simulink model "xfl_ukf2"  (R2015b)
settings: Solver=FixedStepAuto  StartTime=0  StopTime=5  FixedStep=10*(1e-3)  RelTol=1e-3
undefined symbols (not defined in the file or in its folder): qc
libraries: simulink x2
settings Model: Creator=acsl  LastModifiedBy=acsl

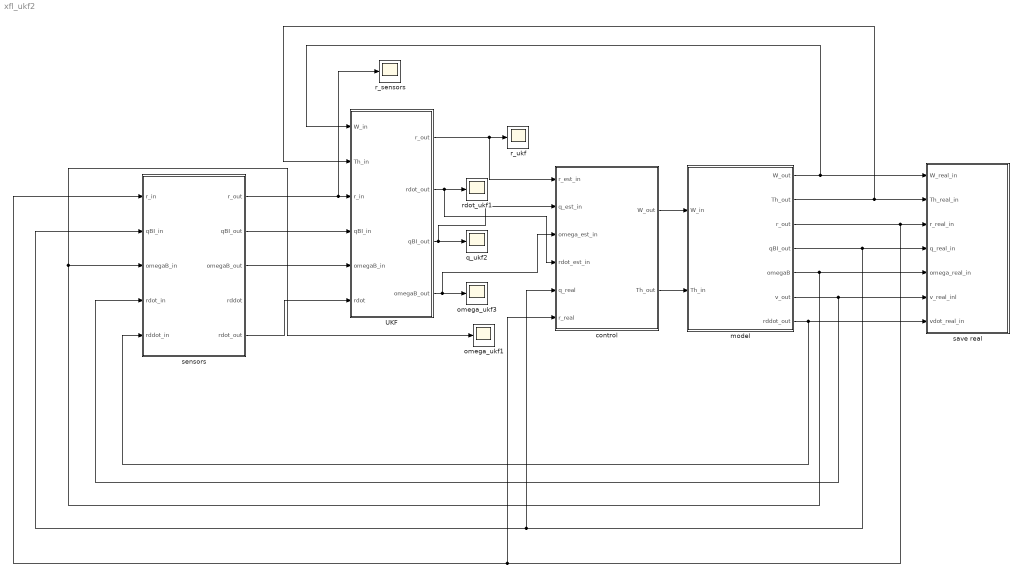
== system xfl_ukf2 ==
  UKF : Subsystem
  control : Subsystem  InitFcn=init
  model : Subsystem
  omega_ukf1 : Scope
  omega_ukf3 : Scope
  q_ukf2 : Scope
  r_sensors : Scope
  r_ukf : Scope
  rdot_ukf1 : Scope
  save real : Subsystem
  sensors : Subsystem
  wires:
  model/2(Th_out) -> UKF/2(Th_in), save real/2(Th_real_in)
  model/7(rddot_out) -> sensors/5(rddot_in), save real/7(vdot_real_in)
  model/5(omegaB) -> sensors/3(omegaB_in), omega_ukf1/1, save real/5(omega_real_in)
  control/1(W_out) -> model/1(W_in)
  control/2(Th_out) -> model/2(Th_in)
  model/3(r_out) -> control/6(r_real), sensors/1(r_in), save real/3(r_real_in)
  model/4(qBI_out) -> sensors/2(qBI_in), control/5(q_real), save real/4(q_real_in)
  model/6(v_out) -> sensors/4(rdot_in), save real/6(v_real_inl)
  model/1(W_out) -> UKF/1(W_in), save real/1(W_real_in)
  sensors/3(omegaB_out) -> UKF/5(omegaB_in)
  sensors/2(qBI_out) -> UKF/4(qBI_in)
  sensors/1(r_out) -> r_sensors/1, UKF/3(r_in)
  UKF/2(rdot_out) -> rdot_ukf1/1, control/4(rdot_est_in)
  UKF/3(qBI_out) -> control/2(q_est_in), q_ukf2/1
  UKF/4(omegaB_out) -> control/3(omega_est_in), omega_ukf3/1
  UKF/1(r_out) -> r_ukf/1, control/1(r_est_in)
  sensors/5(rdot_out) -> UKF/6(rdot)

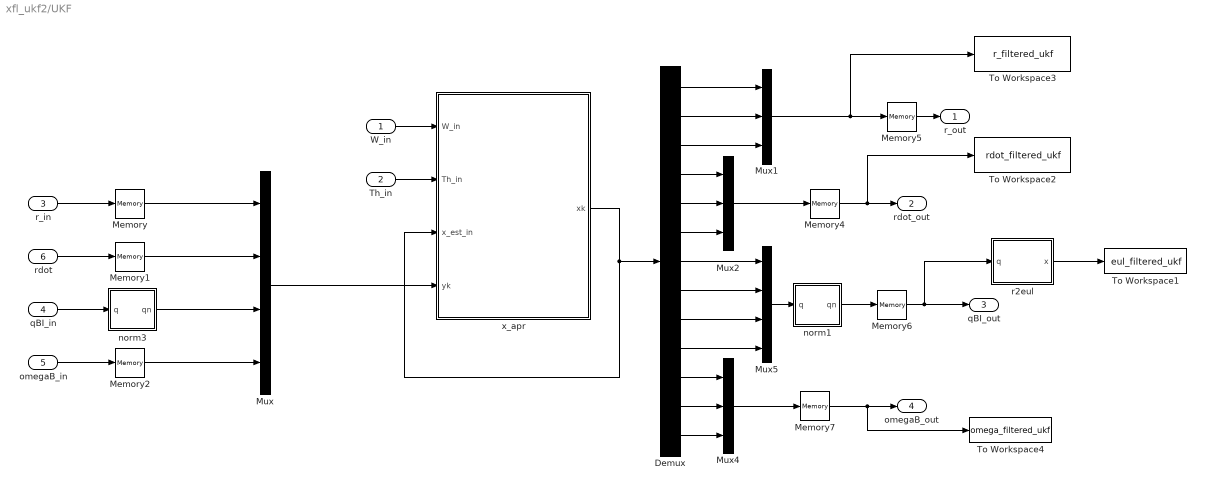
== system xfl_ukf2/UKF ==
  W_in : Inport
  Th_in : Inport  Port=2
  r_in : Inport  Port=3
  qBI_in : Inport  Port=4
  omegaB_in : Inport  Port=5
  rdot : Inport  Port=6
  Demux : Demux  Outputs=13
  Memory : Memory  X0=qc.r0
  Memory{1..2,4,7} (4 alike) : Memory  X0=[0 0 0]'
  Memory5 : Memory  X0=qc.r0
  Memory6 : Memory  X0=qc.qBI0
  Mux : Mux
  Mux1 : Mux  Inputs=3
  Mux2 : Mux  Inputs=3
  Mux4 : Mux  Inputs=3
  Mux5 : Mux
  To Workspace1 : ToWorkspace  VariableName=eul_filtered_ukf  SaveFormat=Timeseries  SampleTime=-1
  To Workspace2 : ToWorkspace  VariableName=rdot_filtered_ukf  SaveFormat=Timeseries  SampleTime=-1
  To Workspace3 : ToWorkspace  VariableName=r_filtered_ukf  SaveFormat=Timeseries  SampleTime=-1
  To Workspace4 : ToWorkspace  VariableName=omega_filtered_ukf  SaveFormat=Timeseries  SampleTime=-1
  norm1 : MATLAB Function  TreatAsAtomicUnit=on
  norm3 : MATLAB Function  TreatAsAtomicUnit=on
  r2eul : MATLAB Function  TreatAsAtomicUnit=on
  x_apr : Subsystem
  r_out : Outport
  rdot_out : Outport  Port=2
  qBI_out : Outport  Port=3
  omegaB_out : Outport  Port=4
  wires:
  qBI_in/1 -> norm3/1(q)
  omegaB_in/1 -> Memory2/1
  rdot/1 -> Memory1/1
  W_in/1 -> x_apr/1(W_in)
  Th_in/1 -> x_apr/2(Th_in)
  Demux/1 -> Mux1/1
  Demux/2 -> Mux1/2
  Demux/3 -> Mux1/3
  Demux/4 -> Mux2/1
  Demux/6 -> Mux2/3
  Demux/5 -> Mux2/2
  Demux/9 -> Mux5/3
  Demux/7 -> Mux5/1
  Demux/8 -> Mux5/2
  Demux/11 -> Mux4/1
  Demux/12 -> Mux4/2
  Demux/13 -> Mux4/3
  Demux/10 -> Mux5/4
  Mux1/1 -> To Workspace3/1, Memory5/1
  Mux2/1 -> Memory4/1
  Mux5/1 -> norm1/1(q)
  r_in/1 -> Memory/1
  norm1/1(qn) -> Memory6/1
  Mux4/1 -> Memory7/1
  r2eul/1(x) -> To Workspace1/1
  Mux/1 -> x_apr/4(yk)
  x_apr/1(xk) -> Demux/1, x_apr/3(x_est_in)
  Memory/1 -> Mux/1
  Memory1/1 -> Mux/2
  Memory2/1 -> Mux/4
  norm3/1(qn) -> Mux/3
  Memory5/1 -> r_out/1
  Memory4/1 -> To Workspace2/1, rdot_out/1
  Memory6/1 -> r2eul/1(q), qBI_out/1
  Memory7/1 -> To Workspace4/1, omegaB_out/1

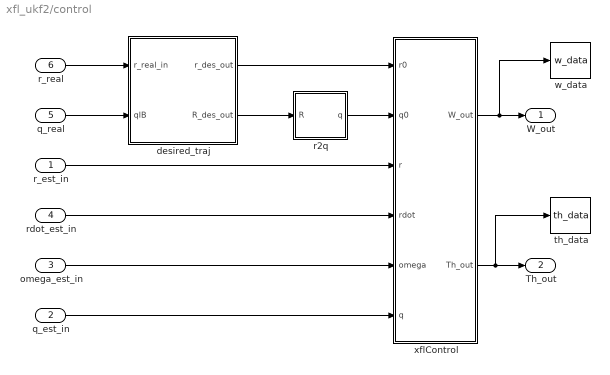
== system xfl_ukf2/control ==
  r_est_in : Inport
  q_est_in : Inport  Port=2
  omega_est_in : Inport  Port=3
  rdot_est_in : Inport  Port=4
  q_real : Inport  Port=5
  r_real : Inport  Port=6
  desired_traj : Subsystem
  r2q : MATLAB Function  TreatAsAtomicUnit=on
  th_data : ToWorkspace  VariableName=th_data  SaveFormat=Timeseries  SampleTime=-1
  w_data : ToWorkspace  VariableName=w_data  SaveFormat=Timeseries  SampleTime=-1
  xflControl : Subsystem
  W_out : Outport
  Th_out : Outport  Port=2
  wires:
  omega_est_in/1 -> xflControl/5(omega)
  q_est_in/1 -> xflControl/6(q)
  rdot_est_in/1 -> xflControl/4(rdot)
  r_est_in/1 -> xflControl/3(r)
  desired_traj/1(r_des_out) -> xflControl/1(r0)
  desired_traj/2(R_des_out) -> r2q/1(R)
  xflControl/1(W_out) -> w_data/1, W_out/1
  xflControl/2(Th_out) -> th_data/1, Th_out/1
  r2q/1(q) -> xflControl/2(q0)
  r_real/1 -> desired_traj/1(r_real_in)
  q_real/1 -> desired_traj/2(qIB)

== system xfl_ukf2/model ==
  W_in : Inport
  Th_in : Inport  Port=2
  draw : Subsystem
  dynamic : Subsystem  StopFcn=close all
  integration : Subsystem
  W_out : Outport
  Th_out : Outport  Port=2
  r_out : Outport  Port=3
  qBI_out : Outport  Port=4
  omegaB : Outport  Port=5
  v_out : Outport  Port=6
  rddot_out : Outport  Port=7
  wires:
  integration/1(r_out) -> dynamic/3(r_in), r_out/1
  dynamic/2(F_I_out) -> integration/2(F_B_in)
  integration/2(qBI_out) -> dynamic/4(q_BI_in), draw/2(qBI), qBI_out/1
  W_in/1 -> W_out/1, dynamic/1(W_in)
  dynamic/1(tau_B_out) -> integration/1(tau_in)
  integration/3(omegaB_out) -> dynamic/5(omegaB_in), omegaB/1
  Th_in/1 -> dynamic/2(Th_in), Th_out/1
  dynamic/3(q_PB_out) -> draw/1(q_PB)
  integration/4(v_out) -> v_out/1
  integration/5(rddot_out) -> rddot_out/1

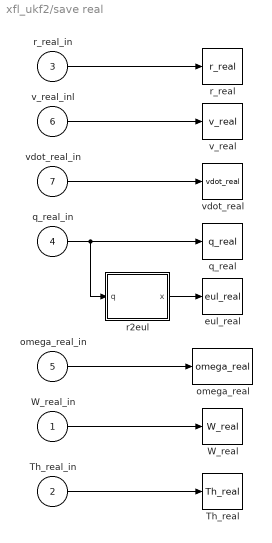
== system xfl_ukf2/save real ==
  W_real_in : Inport
  Th_real_in : Inport  Port=2
  r_real_in : Inport  Port=3
  q_real_in : Inport  Port=4
  omega_real_in : Inport  Port=5
  v_real_inl : Inport  Port=6
  vdot_real_in : Inport  Port=7
  Th_real : ToWorkspace  VariableName=Th_real  SaveFormat=Timeseries  SampleTime=-1
  W_real : ToWorkspace  VariableName=W_real  SaveFormat=Timeseries  SampleTime=-1
  eul_real : ToWorkspace  VariableName=eul_real  SaveFormat=Timeseries  SampleTime=-1
  omega_real : ToWorkspace  VariableName=omega_real  SaveFormat=Timeseries  SampleTime=-1
  q_real : ToWorkspace  VariableName=q_real  SaveFormat=Timeseries  SampleTime=-1
  r2eul : MATLAB Function  TreatAsAtomicUnit=on
  r_real : ToWorkspace  VariableName=r_real  SaveFormat=Timeseries  SampleTime=-1
  v_real : ToWorkspace  VariableName=v_real  SaveFormat=Timeseries  SampleTime=-1
  vdot_real : ToWorkspace  VariableName=vdot_real  SaveFormat=Timeseries  SampleTime=-1
  wires:
  q_real_in/1 -> q_real/1, r2eul/1(q)
  r_real_in/1 -> r_real/1
  v_real_inl/1 -> v_real/1
  vdot_real_in/1 -> vdot_real/1
  r2eul/1(x) -> eul_real/1
  omega_real_in/1 -> omega_real/1
  Th_real_in/1 -> Th_real/1
  W_real_in/1 -> W_real/1

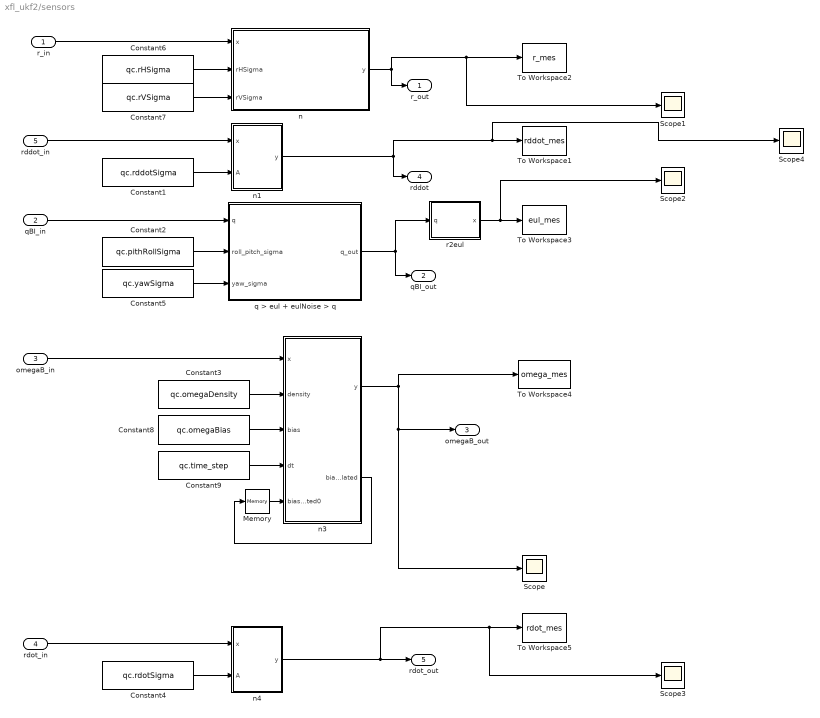
== system xfl_ukf2/sensors ==
  r_in : Inport
  qBI_in : Inport  Port=2
  omegaB_in : Inport  Port=3
  rdot_in : Inport  Port=4
  rddot_in : Inport  Port=5
  Constant1 : Constant  Value=qc.rddotSigma
  Constant2 : Constant  Value=qc.pithRollSigma
  Constant3 : Constant  Value=qc.omegaDensity
  Constant4 : Constant  Value=qc.rdotSigma
  Constant5 : Constant  Value=qc.yawSigma
  Constant6 : Constant  Value=qc.rHSigma
  Constant7 : Constant  Value=qc.rVSigma
  Constant8 : Constant  Value=qc.omegaBias
  Constant9 : Constant  Value=qc.time_step
  Memory : Memory  X0=[0;0;0]
  Scope{,1..4} (5 alike) : Scope
  To Workspace1 : ToWorkspace  VariableName=rddot_mes  SaveFormat=Timeseries  SampleTime=-1
  To Workspace2 : ToWorkspace  VariableName=r_mes  SaveFormat=Timeseries  SampleTime=-1
  To Workspace3 : ToWorkspace  VariableName=eul_mes  SaveFormat=Timeseries  SampleTime=-1
  To Workspace4 : ToWorkspace  VariableName=omega_mes  SaveFormat=Timeseries  SampleTime=-1
  To Workspace5 : ToWorkspace  VariableName=rdot_mes  SaveFormat=Timeseries  SampleTime=-1
  n : MATLAB Function  TreatAsAtomicUnit=on
  n1 : MATLAB Function  TreatAsAtomicUnit=on
  n3 : MATLAB Function  TreatAsAtomicUnit=on
  n4 : MATLAB Function  TreatAsAtomicUnit=on
  q > eul + eulNoise > q : MATLAB Function  TreatAsAtomicUnit=on
  r2eul : MATLAB Function  TreatAsAtomicUnit=on
  r_out : Outport
  qBI_out : Outport  Port=2
  omegaB_out : Outport  Port=3
  rddot : Outport  Port=4
  rdot_out : Outport  Port=5
  wires:
  rddot_in/1 -> n1/1(x)
  qBI_in/1 -> q > eul + eulNoise > q/1(q)
  n3/1(y) -> omegaB_out/1, Scope/1, To Workspace4/1
  q > eul + eulNoise > q/1(q_out) -> qBI_out/1, r2eul/1(q)
  n/1(y) -> Scope1/1, To Workspace2/1, r_out/1
  n1/1(y) -> Scope4/1, To Workspace1/1, rddot/1
  r2eul/1(x) -> Scope2/1, To Workspace3/1
  r_in/1 -> n/1(x)
  Constant6/1 -> n/2(rHSigma)
  Constant1/1 -> n1/2(A)
  Constant2/1 -> q > eul + eulNoise > q/2(roll_pitch_sigma)
  Constant3/1 -> n3/2(density)
  Constant4/1 -> n4/2(A)
  rdot_in/1 -> n4/1(x)
  n4/1(y) -> Scope3/1, To Workspace5/1, rdot_out/1
  Constant5/1 -> q > eul + eulNoise > q/3(yaw_sigma)
  Constant7/1 -> n/3(rVSigma)
  Constant8/1 -> n3/3(bias)
  Constant9/1 -> n3/4(dt)
  Memory/1 -> n3/5(bias_accumulated0)
  n3/2(bias_accumulated) -> Memory/1
  omegaB_in/1 -> n3/1(x)

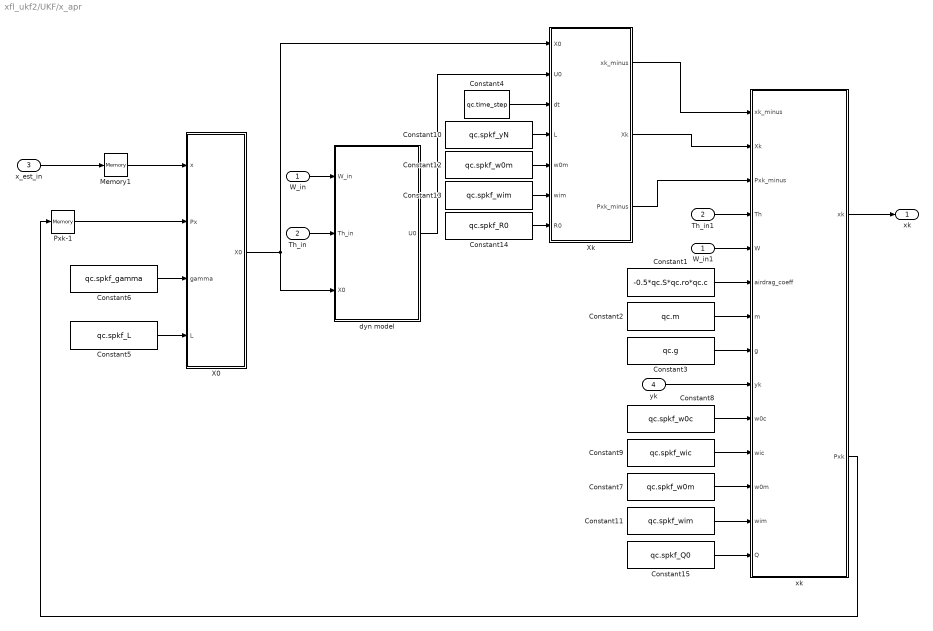
== system xfl_ukf2/UKF/x_apr ==
  W_in : Inport
  Th_in : Inport  Port=2
  x_est_in : Inport  Port=3
  yk : Inport  Port=4
  Constant1 : Constant  Value=-0.5*qc.S*qc.ro*qc.c
  Constant10 : Constant  Value=qc.spkf_yN
  Constant11 : Constant  Value=qc.spkf_wim
  Constant12 : Constant  Value=qc.spkf_w0m
  Constant13 : Constant  Value=qc.spkf_wim
  Constant14 : Constant  Value=qc.spkf_R0
  Constant15 : Constant  Value=qc.spkf_Q0
  Constant2 : Constant  Value=qc.m
  Constant3 : Constant  Value=qc.g
  Constant4 : Constant  Value=qc.time_step
  Constant5 : Constant  Value=qc.spkf_L
  Constant6 : Constant  Value=qc.spkf_gamma
  Constant7 : Constant  Value=qc.spkf_w0m
  Constant8 : Constant  Value=qc.spkf_w0c
  Constant9 : Constant  Value=qc.spkf_wic
  Memory1 : Memory  X0="[0 0 0    0 0 0    1 0 0 0    0 0 0]'"  InheritSampleTime=on
  Pxk-1 : Memory  X0="diag([10 10 10      10 10 10     1e-1 1e-1 1e-1 1e-1    1e-1 1e-1 1e-1])"  InheritSampleTime=on
  Th_in1 : InportShadow  Port=2
  W_in1 : InportShadow
  X0 : MATLAB Function  TreatAsAtomicUnit=on
  Xk : MATLAB Function  TreatAsAtomicUnit=on
  dyn model : Subsystem
  "xk " : MATLAB Function  TreatAsAtomicUnit=on
  xk : Outport
  wires:
  Th_in/1 -> dyn model/2(Th_in)
  W_in/1 -> dyn model/1(W_in)
  x_est_in/1 -> Memory1/1
  Memory1/1 -> X0/1(x)
  X0/1(X0) -> Xk/1(X0), dyn model/3("X0 ")
  dyn model/1(U0) -> Xk/2(U0)
  Constant4/1 -> Xk/3(dt)
  Xk/1(xk_minus) -> "xk "/1(xk_minus)
  Constant1/1 -> "xk "/6(airdrag_coeff)
  Constant2/1 -> "xk "/7(m)
  Constant3/1 -> "xk "/8(g)
  Xk/2(Xk) -> "xk "/2(Xk)
  "xk "/1(xk) -> xk/1
  yk/1 -> "xk "/9(yk)
  Xk/3(Pxk_minus) -> "xk "/3(Pxk_minus)
  Th_in1/1 -> "xk "/4(Th)
  W_in1/1 -> "xk "/5(W)
  Pxk-1/1 -> X0/2(Px)
  "xk "/2(Pxk) -> Pxk-1/1
  Constant5/1 -> X0/4(L)
  Constant6/1 -> X0/3(gamma)
  Constant10/1 -> Xk/4(L)
  Constant12/1 -> Xk/5(w0m)
  Constant13/1 -> Xk/6(wim)
  Constant8/1 -> "xk "/10(w0c)
  Constant9/1 -> "xk "/11(wic)
  Constant7/1 -> "xk "/12(w0m)
  Constant11/1 -> "xk "/13(wim)
  Constant14/1 -> Xk/7(R0)
  Constant15/1 -> "xk "/14(Q)

== system xfl_ukf2/control/desired_traj ==
  r_real_in : Inport
  qIB : Inport  Port=2
  To Workspace1 : ToWorkspace  VariableName=time  SaveFormat=Timeseries  SampleTime=-1
  To Workspace2 : ToWorkspace  VariableName=r_des  SaveFormat=Timeseries  SampleTime=-1
  To Workspace6 : ToWorkspace  VariableName=eul_des  SaveFormat=Timeseries  SampleTime=-1
  dirB : ToWorkspace  VariableName=dirB  SaveFormat=Timeseries  SampleTime=-1
  rFr3 : Scope
  r_target : ToWorkspace  VariableName=r_target  SaveFormat=Timeseries  SampleTime=-1
  time : simulink/Sources/Ramp  slope=1  start=0  X0=0
  traj : MATLAB Function  TreatAsAtomicUnit=on
  r_des_out : Outport
  R_des_out : Outport  Port=2
  wires:
  traj/2(R_des) -> R_des_out/1
  time/1 -> To Workspace1/1, traj/1(t)
  traj/3(eul_des) -> To Workspace6/1
  r_real_in/1 -> traj/2(r)
  traj/1(r_des) -> To Workspace2/1, r_des_out/1
  qIB/1 -> traj/3(qIB)
  traj/4(camera_dir_B) -> dirB/1, rFr3/1
  traj/5(r_target) -> r_target/1

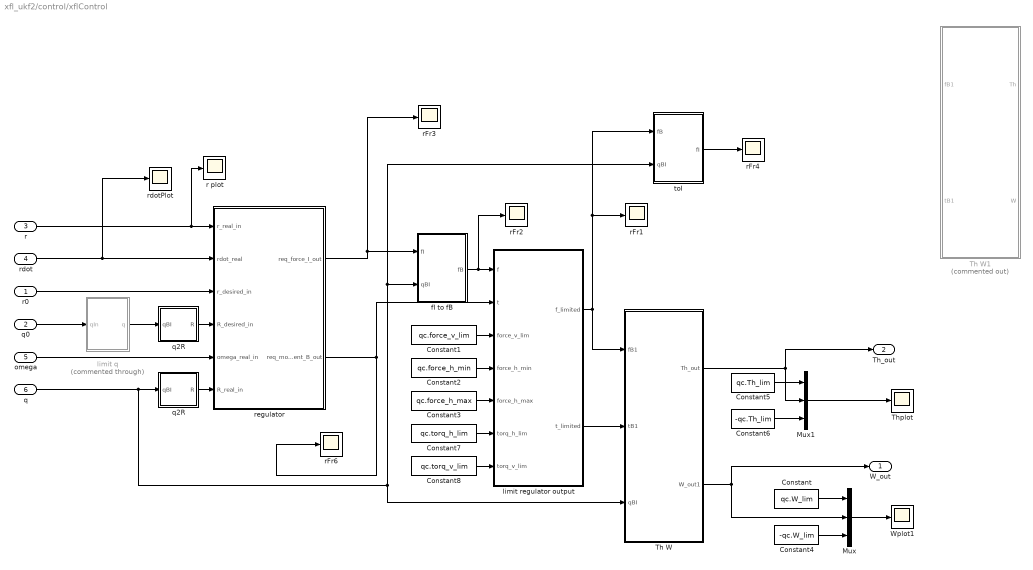
== system xfl_ukf2/control/xflControl ==
  r0 : Inport
  q0 : Inport  Port=2
  r : Inport  Port=3
  rdot : Inport  Port=4
  omega : Inport  Port=5
  q : Inport  Port=6
  Constant : Constant  Value=qc.W_lim
  Constant1 : Constant  Value=qc.force_v_lim
  Constant2 : Constant  Value=qc.force_h_min
  Constant3 : Constant  Value=qc.force_h_max
  Constant4 : Constant  Value=-qc.W_lim
  Constant5 : Constant  Value=qc.Th_lim
  Constant6 : Constant  Value=-qc.Th_lim
  Constant7 : Constant  Value=qc.torq_h_lim
  Constant8 : Constant  Value=qc.torq_v_lim
  Mux : Mux  Inputs=3
  Mux1 : Mux  Inputs=3
  Th W : Subsystem
  Th W1 : Subsystem  Commented=on
  Thplot : Scope
  Wplot1 : Scope
  fI to fB : MATLAB Function  TreatAsAtomicUnit=on
  limit q : MATLAB Function  Commented=through  TreatAsAtomicUnit=on
  limit regulator output : MATLAB Function  TreatAsAtomicUnit=on
  q2R : MATLAB Function  TreatAsAtomicUnit=on
  "q2R " : MATLAB Function  TreatAsAtomicUnit=on
  r plot : Scope
  rFr{1..4,6} (5 alike) : Scope
  rdotPlot : Scope
  regulator : Subsystem
  toI : MATLAB Function  TreatAsAtomicUnit=on
  W_out : Outport
  Th_out : Outport  Port=2
  wires:
  rdot/1 -> rdotPlot/1, regulator/2(rdot_real)
  r0/1 -> regulator/3(r_desired_in)
  r/1 -> r plot/1, regulator/1(r_real_in)
  q0/1 -> limit q/1(qIn)
  omega/1 -> regulator/5(omega_real_in)
  q2R/1(R) -> regulator/6(R_real_in)
  "q2R "/1(R) -> regulator/4(R_desired_in)
  Th W/1(Th_out) -> Th_out/1, Mux1/2
  Th W/2(W_out1) -> Mux/2, W_out/1
  regulator/1(req_force_I_out) -> rFr3/1, fI to fB/1(fI)
  regulator/2(req_moment_B_out) -> rFr6/1, limit regulator output/2(t)
  q/1 -> Th W/3("qBI "), toI/2(qBI), fI to fB/2(qBI), q2R/1(qBI)
  limit q/1(q) -> "q2R "/1(qBI)
  Constant/1 -> Mux/1
  Constant4/1 -> Mux/3
  Mux1/1 -> Thplot/1
  Constant5/1 -> Mux1/1
  Constant6/1 -> Mux1/3
  limit regulator output/2(t_limited) -> Th W/2(tB1)
  limit regulator output/1(f_limited) -> toI/1(fB), rFr1/1, Th W/1(fB1)
  Constant1/1 -> limit regulator output/3(force_v_lim)
  Constant2/1 -> limit regulator output/4(force_h_min)
  Constant3/1 -> limit regulator output/5(force_h_max)
  Constant7/1 -> limit regulator output/6(torq_h_lim)
  Constant8/1 -> limit regulator output/7(torq_v_lim)
  fI to fB/1(fB) -> rFr2/1, limit regulator output/1(f)
  toI/1(fI) -> rFr4/1
  Mux/1 -> Wplot1/1

== system xfl_ukf2/model/draw ==
  q_PB : Inport
  qBI : Inport  Port=2
  Constant : Constant  Value=qc.rays
  Constant1 : Constant  Value=qc.l
  Constant2 : Constant  Value=qc.draw_mode
  Rate Transition : RateTransition
  Rate Transition1 : RateTransition
  draw : MATLAB Function  TreatAsAtomicUnit=on  SystemSampleTime=qc.draw_tick
  wires:
  Constant1/1 -> draw/4(l)
  q_PB/1 -> Rate Transition1/1
  Rate Transition1/1 -> draw/2(q_PB)
  Constant/1 -> draw/3(rays)
  Rate Transition/1 -> draw/1(q_BI)
  qBI/1 -> Rate Transition/1
  Constant2/1 -> draw/5(draw_mode)

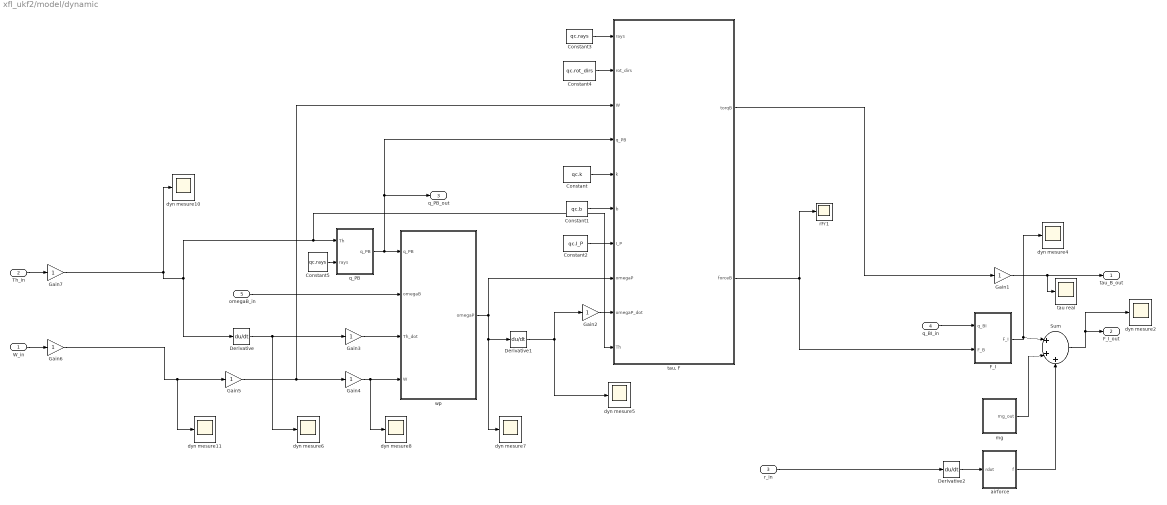
== system xfl_ukf2/model/dynamic ==
  W_in : Inport
  Th_in : Inport  Port=2
  r_in : Inport  Port=3
  q_BI_in : Inport  Port=4
  omegaB_in : Inport  Port=5
  Constant : Constant  Value=qc.k
  Constant1 : Constant  Value=qc.b
  Constant2 : Constant  Value=qc.I_P
  Constant3 : Constant  Value=qc.rays
  Constant4 : Constant  Value=qc.rot_dirs
  Constant5 : Constant  Value=qc.rays
  Derivative : Derivative
  Derivative1 : Derivative
  Derivative2 : Derivative
  F_I : MATLAB Function  TreatAsAtomicUnit=on
  Gain{1..7} (7 alike) : Gain
  Sum : Sum  Inputs=|+++
  airforce : Subsystem
  dyn mesure{2,4..8,10..11} (8 alike) : Scope
  mg : Subsystem
  q_PB : MATLAB Function  TreatAsAtomicUnit=on
  rFr1 : Scope
  tau real : Scope
  "tau, F" : MATLAB Function  TreatAsAtomicUnit=on
  wp : MATLAB Function  TreatAsAtomicUnit=on
  tau_B_out : Outport
  F_I_out : Outport  Port=2
  q_PB_out : Outport  Port=3
  wires:
  q_PB/1(q_PB) -> "tau, F"/4(q_PB), q_PB_out/1, wp/1(q_PB)
  omegaB_in/1 -> wp/2(omegaB)
  Derivative/1 -> dyn mesure6/1, Gain3/1
  wp/1(omegaP) -> dyn mesure7/1, Derivative1/1, "tau, F"/8(omegaP)
  Constant/1 -> "tau, F"/5(k)
  Constant1/1 -> "tau, F"/6(b)
  Constant2/1 -> "tau, F"/7(I_P)
  Constant3/1 -> "tau, F"/1(rays)
  Constant4/1 -> "tau, F"/2(rot_dirs)
  Constant5/1 -> q_PB/2(rays)
  q_BI_in/1 -> F_I/1(q_BI)
  F_I/1(F_I) -> dyn mesure4/1, Sum/1
  mg/1(mg_out) -> Sum/2
  Sum/1 -> dyn mesure2/1, F_I_out/1
  r_in/1 -> Derivative2/1
  airforce/1(f) -> Sum/3
  Derivative2/1 -> airforce/1(rdot)
  Gain2/1 -> "tau, F"/9(omegaP_dot)
  Gain3/1 -> wp/3(Th_dot)
  Gain4/1 -> dyn mesure8/1, wp/4(W)
  Derivative1/1 -> dyn mesure5/1, Gain2/1
  Gain1/1 -> tau_B_out/1, tau real/1
  Gain5/1 -> "tau, F"/3(W), Gain4/1
  Gain6/1 -> dyn mesure11/1, Gain5/1
  Gain7/1 -> "tau, F"/10(Th), q_PB/1(Th), Derivative/1, dyn mesure10/1
  W_in/1 -> Gain6/1
  Th_in/1 -> Gain7/1
  "tau, F"/1(torqB) -> Gain1/1
  "tau, F"/2(forceB) -> rFr1/1, F_I/2(F_B)

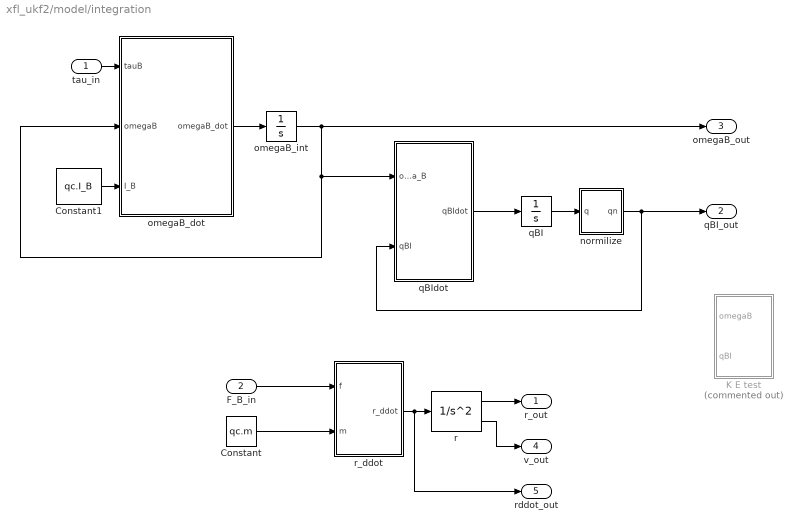
== system xfl_ukf2/model/integration ==
  tau_in : Inport
  F_B_in : Inport  Port=2
  Constant : Constant  Value=qc.m
  Constant1 : Constant  Value=qc.I_B
  K E test : Subsystem  Commented=on
  normilize : MATLAB Function  TreatAsAtomicUnit=on
  omegaB_dot : MATLAB Function  TreatAsAtomicUnit=on
  omegaB_int : Integrator  InitialCondition=qc.omegaB0
  qBI : Integrator  InitialCondition=qc.qBI0
  qBIdot : MATLAB Function  TreatAsAtomicUnit=on
  r : SecondOrderIntegrator  ICX=qc.r0  ICDXDT=qc.v0
  r_ddot : MATLAB Function  TreatAsAtomicUnit=on
  r_out : Outport
  qBI_out : Outport  Port=2
  omegaB_out : Outport  Port=3
  v_out : Outport  Port=4
  rddot_out : Outport  Port=5
  wires:
  r/1 -> r_out/1
  r_ddot/1(r_ddot) -> rddot_out/1, r/1
  Constant/1 -> r_ddot/2(m)
  omegaB_int/1 -> omegaB_out/1, qBIdot/1(omega_B), omegaB_dot/2(omegaB)
  Constant1/1 -> omegaB_dot/3(I_B)
  tau_in/1 -> omegaB_dot/1(tauB)
  qBIdot/1(qBIdot) -> qBI/1
  qBI/1 -> normilize/1(q)
  normilize/1(qn) -> qBI_out/1, qBIdot/2(qBI)
  F_B_in/1 -> r_ddot/1(f)
  omegaB_dot/1(omegaB_dot) -> omegaB_int/1
  r/2 -> v_out/1

== system xfl_ukf2/UKF/x_apr/dyn model ==
  W_in : Inport
  Th_in : Inport  Port=2
  "X0 " : Inport  Port=3
  Constant1 : Constant  Value=qc.I_B
  Constant2 : Constant  Value=qc.g
  Constant3 : Constant  Value=-0.5*qc.S*qc.ro*qc.c
  Constant5 : Constant  Value=qc.m
  simple model : MATLAB Function  TreatAsAtomicUnit=on
  U0 : Outport
  wires:
  simple model/1(U0) -> U0/1
  Th_in/1 -> simple model/1(Th)
  W_in/1 -> simple model/2(W)
  "X0 "/1 -> simple model/3(Xs)
  Constant5/1 -> simple model/4(m)
  Constant1/1 -> simple model/6(I)
  Constant2/1 -> simple model/5(g)
  Constant3/1 -> simple model/7(airdrag_coeff)

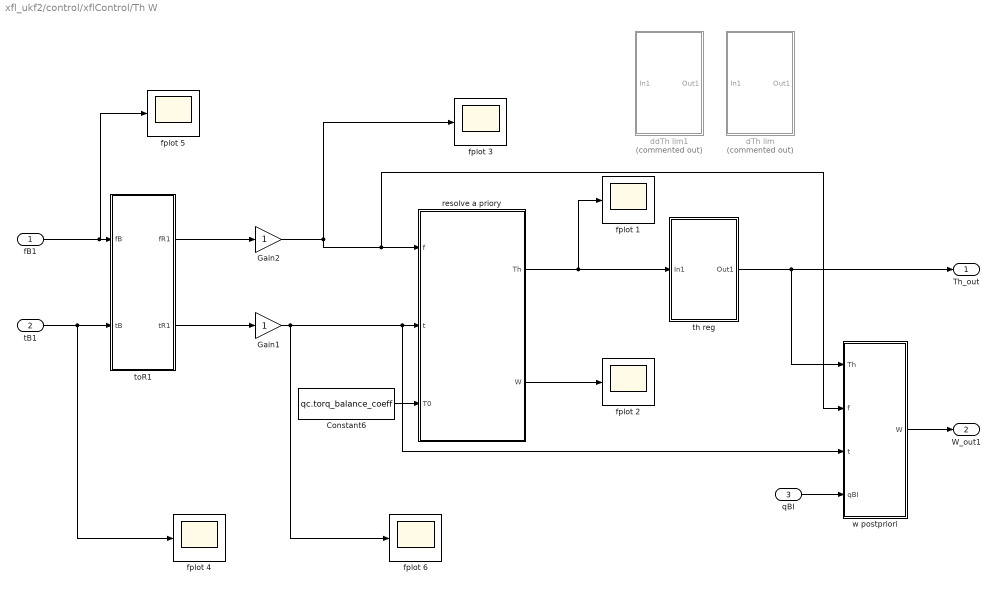
== system xfl_ukf2/control/xflControl/Th W ==
  fB1 : Inport
  tB1 : Inport  Port=2
  "qBI " : Inport  Port=3
  Constant6 : Constant  Value=qc.torq_balance_coeff
  Gain1 : Gain
  Gain2 : Gain
  dTh lim : Subsystem  Commented=on
  ddTh lim1 : Subsystem  Commented=on
  fplot {1..6} (6 alike) : Scope
  resolve a priory : MATLAB Function  TreatAsAtomicUnit=on
  th reg : Subsystem
  toR1 : MATLAB Function  TreatAsAtomicUnit=on
  w postpriori : MATLAB Function  TreatAsAtomicUnit=on
  Th_out : Outport
  W_out1 : Outport  Port=2
  wires:
  Gain1/1 -> w postpriori/3(t), resolve a priory/2(t), fplot 6/1
  Gain2/1 -> fplot 3/1, w postpriori/2(f), resolve a priory/1(f)
  Constant6/1 -> resolve a priory/3(T0)
  fB1/1 -> fplot 5/1, toR1/1(fB)
  toR1/2(tR1) -> Gain1/1
  toR1/1(fR1) -> Gain2/1
  w postpriori/1(W) -> W_out1/1
  th reg/1(Out1) -> Th_out/1, w postpriori/1(Th)
  resolve a priory/1(Th) -> fplot 1/1, th reg/1(In1)
  "qBI "/1 -> w postpriori/4(qBI)
  resolve a priory/2(W) -> fplot 2/1
  tB1/1 -> fplot 4/1, toR1/2(tB)

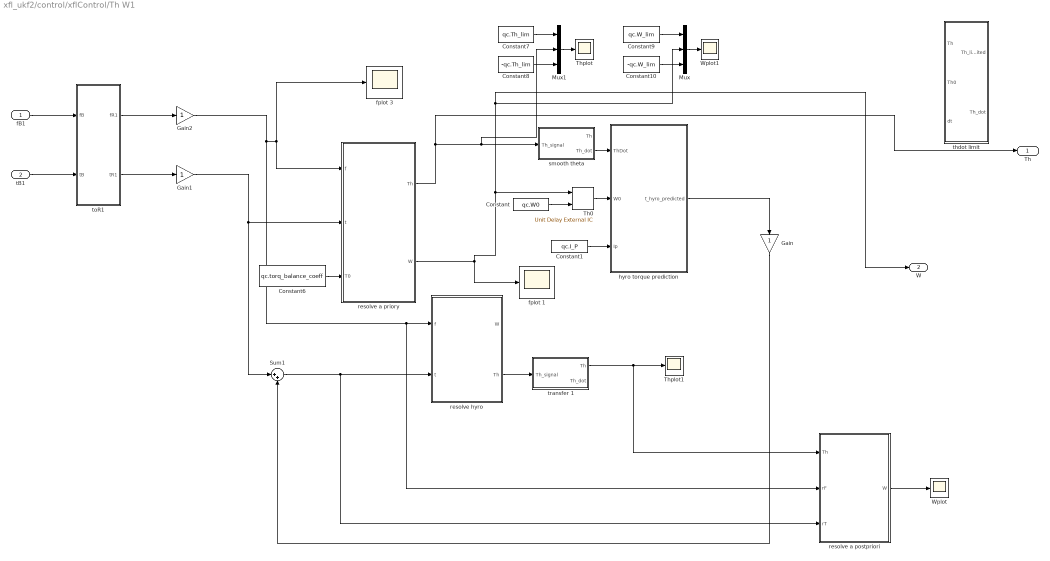
== system xfl_ukf2/control/xflControl/Th W1 ==
  fB1 : Inport
  tB1 : Inport  Port=2
  Constant : Constant  Value=qc.W0
  Constant1 : Constant  Value=qc.I_P
  Constant10 : Constant  Value=-qc.W_lim
  Constant6 : Constant  Value=qc.torq_balance_coeff
  Constant7 : Constant  Value=qc.Th_lim
  Constant8 : Constant  Value=-qc.Th_lim
  Constant9 : Constant  Value=qc.W_lim
  Gain : Gain
  Gain1 : Gain
  Gain2 : Gain
  Mux : Mux  Inputs=3
  Mux1 : Mux  Inputs=3
  Sum1 : Sum  Inputs=|++
  Th0 : simulink/Additional Math & Discrete/Additional Discrete/Unit Delay External IC  tsamp=-1
  Thplot : Scope
  Thplot1 : Scope
  Wplot : Scope
  Wplot1 : Scope
  fplot 1 : Scope
  fplot 3 : Scope
  hyro torque prediction : MATLAB Function  TreatAsAtomicUnit=on
  resolve a postpriori : MATLAB Function  TreatAsAtomicUnit=on
  resolve a priory : MATLAB Function  TreatAsAtomicUnit=on
  resolve hyro : Subsystem
  smooth theta : Subsystem
  thdot limit : MATLAB Function  TreatAsAtomicUnit=on
  toR1 : MATLAB Function  TreatAsAtomicUnit=on
  transfer 1 : Subsystem
  Th : Outport
  W : Outport  Port=2
  wires:
  toR1/1(fR1) -> Gain2/1
  toR1/2(tR1) -> Gain1/1
  fB1/1 -> toR1/1(fB)
  tB1/1 -> toR1/2(tB)
  Constant10/1 -> Mux/3
  Mux/1 -> Wplot1/1
  Constant9/1 -> Mux/1
  resolve a priory/2(W) -> fplot 1/1, Th0/1, Mux/2, W/1
  Constant8/1 -> Mux1/3
  Constant7/1 -> Mux1/1
  Mux1/1 -> Thplot/1
  resolve a priory/1(Th) -> smooth theta/1(Th_signal), Mux1/2, Th/1
  Constant6/1 -> resolve a priory/3(T0)
  resolve a postpriori/1(W) -> Wplot/1
  Sum1/1 -> resolve a postpriori/3(rT), resolve hyro/2(t)
  transfer 1/1(Th) -> Thplot1/1, resolve a postpriori/1(Th)
  Gain2/1 -> resolve a priory/1(f), fplot 3/1, resolve hyro/1(f), resolve a postpriori/2(rF)
  Gain1/1 -> Sum1/1, resolve a priory/2(t)
  Gain/1 -> Sum1/2
  resolve hyro/2(Th) -> transfer 1/1(Th_signal)
  hyro torque prediction/1(t_hyro_predicted) -> Gain/1
  smooth theta/2(Th_dot) -> hyro torque prediction/1(ThDot)
  Constant1/1 -> hyro torque prediction/3(Ip)
  Constant/1 -> Th0/2
  Th0/1 -> hyro torque prediction/2(W0)

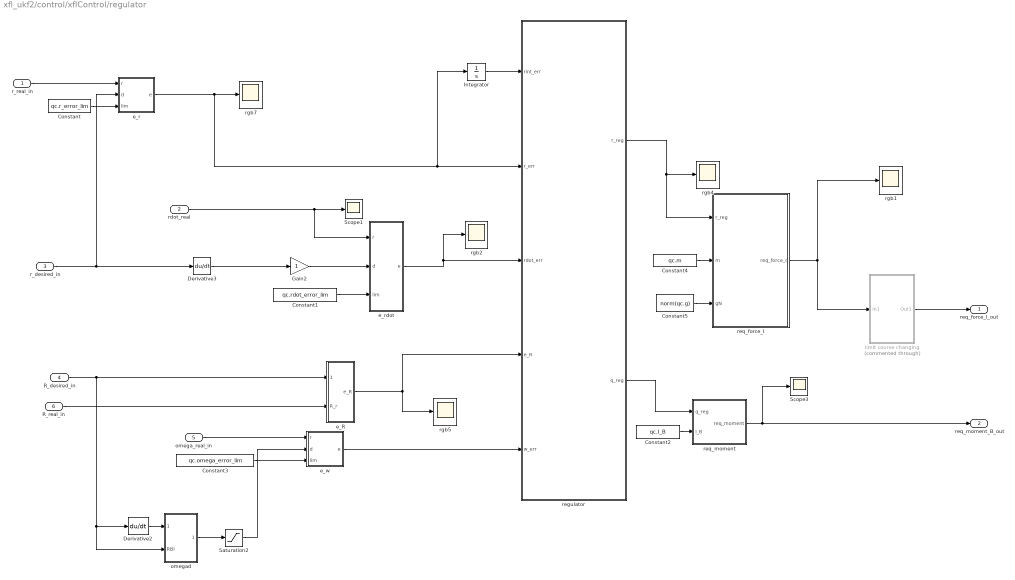
== system xfl_ukf2/control/xflControl/regulator ==
  r_real_in : Inport
  rdot_real : Inport  Port=2
  r_desired_in : Inport  Port=3
  R_desired_in : Inport  Port=4
  omega_real_in : Inport  Port=5
  R_real_in : Inport  Port=6
  Constant : Constant  Value=qc.r_error_lim
  Constant1 : Constant  Value=qc.rdot_error_lim
  Constant2 : Constant  Value=qc.I_B
  Constant3 : Constant  Value=qc.omega_error_lim
  Constant4 : Constant  Value=qc.m
  Constant5 : Constant  Value=norm(qc.g)
  Derivative2 : Derivative
  Derivative3 : Derivative
  Gain2 : Gain
  Integrator : Integrator
  Saturation2 : Saturate  UpperLimit=qc.w_des_lim  LowerLimit=-qc.w_des_lim
  Scope1 : Scope
  Scope3 : Scope
  e_R : MATLAB Function  TreatAsAtomicUnit=on
  e_r : MATLAB Function  TreatAsAtomicUnit=on
  e_rdot : MATLAB Function  TreatAsAtomicUnit=on
  e_w : MATLAB Function  TreatAsAtomicUnit=on
  limit course changing : Subsystem  Commented=through
  omegad : MATLAB Function  TreatAsAtomicUnit=on
  regulator : MATLAB Function  TreatAsAtomicUnit=on
  req_force_I : MATLAB Function  TreatAsAtomicUnit=on
  req_moment : MATLAB Function  TreatAsAtomicUnit=on
  rgb{1..2,4..5,7} (5 alike) : Scope
  req_force_I_out : Outport
  req_moment_B_out : Outport  Port=2
  wires:
  R_real_in/1 -> e_R/2(R_r)
  Derivative3/1 -> Gain2/1
  Saturation2/1 -> e_w/2(d)
  r_desired_in/1 -> e_r/2(d), Derivative3/1
  r_real_in/1 -> e_r/1(r)
  Constant3/1 -> e_w/3(lim)
  omega_real_in/1 -> e_w/1(r)
  e_w/1(e) -> regulator/5(w_err)
  Constant1/1 -> e_rdot/3(lim)
  rdot_real/1 -> Scope1/1, e_rdot/1(r)
  e_rdot/1(e) -> rgb2/1, regulator/3(rdot_err)
  Constant/1 -> e_r/3(lim)
  e_r/1(e) -> rgb7/1, regulator/2(r_err), Integrator/1
  e_R/1(e_R) -> rgb5/1, regulator/4(e_R)
  omegad/1(omega) -> Saturation2/1
  R_desired_in/1 -> e_R/1(R_d), Derivative2/1, omegad/2(RBI)
  Derivative2/1 -> omegad/1(RBIdot)
  regulator/2(q_reg) -> req_moment/1(q_reg)
  req_moment/1(req_moment) -> Scope3/1, req_moment_B_out/1
  Constant2/1 -> req_moment/2(I_B)
  regulator/1(r_reg) -> req_force_I/1(r_reg), rgb4/1
  req_force_I/1(req_force_I) -> limit course changing/1(In1), rgb1/1
  Constant4/1 -> req_force_I/2(m)
  Constant5/1 -> req_force_I/3(gN)
  Gain2/1 -> e_rdot/2(d)
  Integrator/1 -> regulator/1(rint_err)
  limit course changing/1(Out1) -> req_force_I_out/1

== system xfl_ukf2/model/dynamic/airforce ==
  rdot : Inport
  Constant10 : Constant  Value=qc.S
  Constant8 : Constant  Value=qc.ro
  Constant9 : Constant  Value=qc.c
  air force I : MATLAB Function  TreatAsAtomicUnit=on
  f : Outport
  wires:
  air force I/1(f) -> f/1
  Constant9/1 -> air force I/3(c)
  Constant10/1 -> air force I/4(S)
  Constant8/1 -> air force I/2(ro)
  rdot/1 -> air force I/1(r_dot)

== system xfl_ukf2/model/dynamic/mg ==
  Constant6 : Constant  Value=qc.m
  Constant7 : Constant  Value=qc.g
  mg : MATLAB Function  TreatAsAtomicUnit=on
  mg_out : Outport
  wires:
  Constant7/1 -> mg/2(g)
  Constant6/1 -> mg/1(m)
  mg/1(mg) -> mg_out/1

== system xfl_ukf2/model/integration/K E test ==
  omegaB : Inport
  qBI : Inport  Port=2
  Constant2 : Constant  Value=qc.I_B
  "K, E" : MATLAB Function  TreatAsAtomicUnit=on
  rgb : Scope
  rgb1 : Scope
  wires:
  omegaB/1 -> "K, E"/2(omega_B)
  qBI/1 -> "K, E"/3(qBI)
  "K, E"/1(K) -> rgb/1
  "K, E"/2(E) -> rgb1/1
  Constant2/1 -> "K, E"/1(I_B)

== system xfl_ukf2/control/xflControl/Th W/dTh lim ==
  In1 : Inport
  Constant1 : Constant  Value=1e-2
  Memory : Memory  X0=[0 0 0 0]'
  fplot 1 : Scope
  thdot limit : MATLAB Function  TreatAsAtomicUnit=on
  Out1 : Outport
  wires:
  thdot limit/2(Th_dot) -> fplot 1/1
  Memory/1 -> thdot limit/2(Th0)
  thdot limit/1(Th_limited) -> Out1/1
  Constant1/1 -> thdot limit/3(dt)
  In1/1 -> thdot limit/1(Th), Memory/1

== system xfl_ukf2/control/xflControl/Th W/ddTh lim1 ==
  In1 : Inport
  Constant1 : Constant  Value=1e-2
  Memory : Memory  X0=[0 0 0 0]'
  Memory1 : Memory  X0=[0 0 0 0]'
  fplot {1..4} (4 alike) : Scope
  thdot limit : MATLAB Function  TreatAsAtomicUnit=on
  Out1 : Outport
  wires:
  thdot limit/3(ddTh) -> fplot 2/1
  Memory1/1 -> thdot limit/2(Th1), Memory/1
  thdot limit/2(dTh1_limited) -> fplot 1/1
  Memory/1 -> thdot limit/3(Th0)
  thdot limit/1(Th_limited) -> Out1/1, fplot 3/1, Memory1/1
  Constant1/1 -> thdot limit/4(dt)
  In1/1 -> thdot limit/1(Th2), fplot 4/1

== system xfl_ukf2/control/xflControl/Th W/th reg ==
  In1 : Inport
  Derivative : Derivative
  Memory1 : Memory  X0=[0 0 0 0]'
  fplot 1 : Scope
  fplot 3 : Scope
  fplot 4 : Scope
  thdot limit : MATLAB Function  TreatAsAtomicUnit=on
  Out1 : Outport
  wires:
  In1/1 -> thdot limit/1(Th_des), fplot 4/1
  Memory1/1 -> thdot limit/2(Th0)
  thdot limit/1(Th) -> Derivative/1, Memory1/1, Out1/1, fplot 3/1
  Derivative/1 -> fplot 1/1

== system xfl_ukf2/control/xflControl/Th W1/resolve hyro ==
  f : Inport
  t : Inport  Port=2
  Constant6 : Constant  Value=qc.b
  Constant7 : Constant  Value=qc.k
  Constant8 : Constant  Value=qc.g
  Constant9 : Constant  Value=qc.m
  resolve hyro : MATLAB Function  TreatAsAtomicUnit=on
  W : Outport
  Th : Outport  Port=2
  wires:
  f/1 -> resolve hyro/1(f)
  t/1 -> resolve hyro/2(t)
  Constant7/1 -> resolve hyro/5(k)
  Constant9/1 -> resolve hyro/3(m)
  Constant8/1 -> resolve hyro/4(gV)
  resolve hyro/2(Th) -> Th/1
  resolve hyro/1(W) -> W/1
  Constant6/1 -> resolve hyro/6(b)

== system xfl_ukf2/control/xflControl/Th W1/smooth theta ==
  Th_signal : Inport
  Demux : Demux
  Derivative : Derivative
  Mux : Mux
  Transfer Fcn{,1..3} (4 alike) : TransferFcn  Numerator=qc.Th_transfer_top  Denominator=qc.Th_transfer_bot
  Th : Outport
  Th_dot : Outport  Port=2
  wires:
  Derivative/1 -> Th_dot/1
  Th_signal/1 -> Demux/1
  Mux/1 -> Th/1, Derivative/1
  Transfer Fcn3/1 -> Mux/4
  Transfer Fcn2/1 -> Mux/3
  Transfer Fcn1/1 -> Mux/2
  Demux/4 -> Transfer Fcn3/1
  Demux/3 -> Transfer Fcn2/1
  Demux/2 -> Transfer Fcn1/1
  Transfer Fcn/1 -> Mux/1
  Demux/1 -> Transfer Fcn/1

== system xfl_ukf2/control/xflControl/Th W1/transfer 1 ==
  Th_signal : Inport
  Demux : Demux
  Derivative : Derivative
  Mux : Mux
  Transfer Fcn{,1..3} (4 alike) : TransferFcn  Numerator=qc.Th_transfer_top  Denominator=qc.Th_transfer_bot
  Th : Outport
  Th_dot : Outport  Port=2
  wires:
  Demux/1 -> Transfer Fcn/1
  Transfer Fcn/1 -> Mux/1
  Demux/2 -> Transfer Fcn1/1
  Demux/3 -> Transfer Fcn2/1
  Demux/4 -> Transfer Fcn3/1
  Transfer Fcn1/1 -> Mux/2
  Transfer Fcn2/1 -> Mux/3
  Transfer Fcn3/1 -> Mux/4
  Mux/1 -> Derivative/1, Th/1
  Th_signal/1 -> Demux/1
  Derivative/1 -> Th_dot/1

== system xfl_ukf2/control/xflControl/regulator/limit course changing ==
  In1 : Inport
  Memory : Memory  X0=[0 0 0]'
  limit course changing : MATLAB Function  TreatAsAtomicUnit=on
  Out1 : Outport
  wires:
  In1/1 -> limit course changing/1(x1)
  Memory/1 -> limit course changing/2(x0)
  limit course changing/1(x) -> Out1/1, Memory/1

== matlab function xfl_ukf2/model/dynamic/wp ==
  data: q_PB input; omegaP output; omegaB input; Th_dot input; W input
function omegaP  = fcn(q_PB, omegaB, Th_dot, W)

omegaP = zeros(4*3,1);
for i = 1:4
    q_pb = q_PB(:, i);
    q_bp = quatDual(q_pb);
    w = sign(W(i))*sqrt(abs(W(i)));
    omegaP(3*i-2:3*i, 1) = quatRotate(q_bp, omegaB) + [Th_dot(i); 0; w];
end

== matlab function xfl_ukf2/model/integration/normilize ==
  data: q input; qn output
function qn  = fcn(q)
qn = q / norm(q);

== matlab function xfl_ukf2/model/dynamic/tau, F ==
  data: torqB output; forceB output; rays input; rot_dirs input; W input; q_PB input; k input; b input; I_P input; omegaP input; omegaP_dot input; Th input
function [torqB, forceB]= fcn(rays, rot_dirs, W, q_PB, k, b, I_P, omegaP, omegaP_dot, Th)

torqB = [0;0;0];
forceB = [0;0;0];

for i = 1:4
    ray = rays(3*i-2:3*i);
    dir = rot_dirs(i);  
    omega_p = omegaP(3*i-2:3*i);
    omega_pz = omega_p(3);
    omega_p_dot = omegaP_dot(3*i-2:3*i);
    q_pb = q_PB(:, i);

    fp = dir * [0;0;k*W(i)];
    fb = quatRotate(q_pb, fp);
        
    tau_p_ext = [0;0;-b*abs(omega_pz)*omega_pz];
    n = 1; %%%%%%% 1 !!!!!!!!!!!!
    tau_p = n*I_P*omega_p_dot + n*cross(omega_p, I_P*omega_p) - tau_p_ext;
    tau_b = cross(ray, fb) - quatRotate(q_pb, tau_p);
    
    torqB = torqB + tau_b;  
    forceB = forceB + fb;
end


% % simple dynamic modeling
% J = xfl_J_B(Th(1),Th(2),Th(3),Th(4));
% xdyn = J*W;
% f = xdyn(1:3);
% t = xdyn(4:6);

== matlab function xfl_ukf2/control/xflControl/regulator/e_R ==
  data: R_d input; R_r input; e_R output size=3
function e_R = e_r(R_d, R_r)
Me_R = R_r'*R_d - R_d'*R_r;
e_R = 0.5*[-Me_R(2,3); Me_R(1,3); -Me_R(1,2)];
end

== matlab function xfl_ukf2/model/dynamic/mg/mg ==
  data: m input; mg output; g input
function mg  = fcn(m, g)
mg = m*g;

== matlab function xfl_ukf2/model/integration/r_ddot ==
  data: r_ddot output; f input; m input
function r_ddot  = fcn(f, m)

r_ddot = f/m;

== matlab function xfl_ukf2/save real/r2eul ==
  data: q input; x output
function x = fnc(q)
eul = quat2eul(q');
x = eul';
end

== matlab function xfl_ukf2/model/integration/omegaB_dot ==
  data: tauB input; omegaB_dot output; omegaB input; I_B input
function omegaB_dot  = fcn(tauB, omegaB, I_B)
omegaB_dot = I_B^(-1) * (tauB - 1*cross(omegaB, I_B * omegaB));

== matlab function xfl_ukf2/model/dynamic/F_I ==
  data: q_BI input; F_I output; F_B input
function F_I  = fcn(q_BI, F_B)
F_I = quatRotate(q_BI, F_B);

== matlab function xfl_ukf2/model/integration/qBIdot ==
  data: omega_B input; qBIdot output; qBI input
function qBIdot  = fcn(omega_B, qBI)
qw = [0;omega_B];
qBIdot = 0.5*quatMultiply(qBI, qw);

== matlab function xfl_ukf2/control/xflControl/regulator/e_r ==
  data: r input; d input; e output size=3; lim input
function e = e_r(r, d, lim)
e = d - r;
n = norm(e);
if n < lim
    return;
end
e = lim*e/n;
end

== matlab function xfl_ukf2/model/draw/draw ==
  data: q_BI input; q_PB input; rays input; l input; draw_mode input
function drawFly(q_BI, q_PB, rays, l, draw_mode)
drawFly(q_BI, q_PB, rays, l, draw_mode)
end

== matlab function xfl_ukf2/model/integration/K E test/K, E ==
  data: I_B input; omega_B input; qBI input; K output; E output
function [K, E] = fcn(I_B, omega_B, qBI)
K_B = I_B*omega_B;
K = quatRotate(qBI, K_B);
E = omega_B'*I_B*omega_B / 2;

== matlab function xfl_ukf2/control/xflControl/regulator/e_rdot ==
  data: r input; d input; e output size=3; lim input
function e = e_r(r, d, lim)
e = d - r;
n = norm(e);
if n < lim
    return;
end
e = lim*e/n;
end

== matlab function xfl_ukf2/control/xflControl/regulator/e_w ==
  data: r input; d input; e output size=3; lim input
function e = e_r(r, d, lim)
e = d - r;
n = norm(e);
if n < lim
    return;
end
e = lim*e/n;
end

== matlab function xfl_ukf2/control/xflControl/regulator/regulator ==
  data: rint_err input; r_err input; rdot_err input; r_reg output; e_R input; w_err input; q_reg output
function [r_reg, q_reg]= x_e(rint_err, r_err, rdot_err, e_R, w_err)
 
% if norm(r_err) < 0.2
%     r_err = zeros(3,1);
% end
% 
% if norm(rdot_err) < 0.1
%     rdot_err = zeros(3,1);
% end
% 
% if norm(e_R) < 0.02
%     e_R = zeros(3,1);
% end
% 
% if norm(w_err) < 0.05
%     w_err = zeros(3,1);
% end

Dr = [10,0,0;
      0,10,0;
      0,0,10]*2;

Pr =   [10,0,0;
       0,10,0;
       0,0,8]*2;
   
Ir =  [1,0,0;
       0,1,0;
       0,0,3]*2;
   
int_lim = 3;
rint_err = min(max(rint_err, -int_lim), int_lim);
 
r_reg =  Dr*(rdot_err)+ Pr*(r_err) + Ir*rint_err;

Dq =   [1,0,0;
        0,1,0;
        0,0,1]*8;

Pq =   [1,0,0; 
        0,1,0;
        0,0,1]*8;
          
q_reg = Dq*(w_err) + Pq*(e_R);
end

== matlab function xfl_ukf2/control/xflControl/regulator/omegad ==
  data: omega output; RBIdot input; RBI input
function omega  = fcn(RBIdot, RBI)

R = RBI'*RBIdot;
omega = [-R(2,3); R(1,3); -R(1,2)];

== matlab function xfl_ukf2/control/xflControl/q2R ==
  data: qBI input; R output
function R = q2R(qBI)
R = quat2matrix(qBI);
end

== matlab function xfl_ukf2/control/xflControl/limit regulator output ==
  data: f_limited output; f input; t_limited output; t input; force_v_lim input; force_h_min input; force_h_max input; torq_h_lim input; torq_v_lim input
function [f_limited,t_limited]= fcn(f, t, force_v_lim, force_h_min, force_h_max, torq_h_lim, torq_v_lim)

q = [cos(pi/4/2) 0 0 -sin(pi/4/2)]';
f = quatRotate(q, f);
t = quatRotate(q, t);

f_limited = zeros(3,1);
t_limited = zeros(3,1);

f_limited(1) = set_between(f(1), force_v_lim, -force_v_lim);
f_limited(2) = set_between(f(2), force_v_lim, -force_v_lim);
f_limited(3) = set_between(f(3), force_h_max, force_h_min);

t_limited(1) = set_between(t(1), torq_h_lim, -torq_h_lim);
t_limited(2) = set_between(t(2), torq_h_lim, -torq_h_lim);
t_limited(3) = set_between(t(3), torq_v_lim, -torq_v_lim);


q = [cos(pi/4/2) 0 0 sin(pi/4/2)]';
f_limited = quatRotate(q, f_limited);
t_limited = quatRotate(q, t_limited);

end

== matlab function xfl_ukf2/control/xflControl/q2R  ==
  data: qBI input; R output
function R = q2R(qBI)
R = quat2matrix(qBI);
end

== matlab function xfl_ukf2/control/xflControl/fI to fB ==
  data: fI input; qBI input; fB output
function fB = q2R(fI, qBI)
qIB = quatDual(qBI);
fB = quatRotate(qIB, fI);
end

== matlab function xfl_ukf2/control/xflControl/Th W/toR1 ==
  data: fB input; fR1 output; tB input; tR1 output
function [fR1, tR1]= fcn(fB, tB)
q = [cos(pi/4/2) 0 0 -sin(pi/4/2)]';
fR1 = quatRotate(q, fB);
tR1 = quatRotate(q, tB);
end

== matlab function xfl_ukf2/control/r2q ==
  data: R input; q output
function q = q2R(R)
q = matrix2quat(R);
end

== matlab function xfl_ukf2/sensors/r2eul ==
  data: q input; x output
function x = fnc(q)
q = q / norm(q);
eul = quat2eul(q');
x = eul';
end

== matlab function xfl_ukf2/control/desired_traj/traj ==
  data: r_des output; R_des output; t input; eul_des output; r input; qIB input; camera_dir_B output; r_target output
function [r_des, R_des, eul_des, camera_dir_B, r_target] = curve(t, r, qIB)
r_aim0 = 1*[2, 50, 5]';
A = 30;
T = 120;

t1 = min(inf, t);
r_aim = r_aim0 + [1.7*A*sin(2*pi*t1/T) , -1.0*A*cos(2*pi*t1/T), 2*sqrt(t1) - 5 * sin(2*pi*t1/2/T)]';

r_des = r_aim;

r_target0 = 0.5*[100, 40, -15]';
r_target = r_target0 + [2*A*sin(2*pi*t/T) , -2.5*A*cos(2*pi*t/T), 2*sqrt(t) + 2 * sin(2*pi*t/40) + 3 * sin(2*pi*t/50)]';
q = quatBetweenVectors([1 0 0]', r_target-r);
R_des = quat2rotm(q');
eul_des = quat2eul(q')';

camera_dir_B = quatRotate(quatDual(qIB), r_target-r);
camera_dir_B = camera_dir_B / norm(camera_dir_B);
camera_dir_B = camera_dir_B .* [0 1 1]';

end

== matlab function xfl_ukf2/model/dynamic/q_PB ==
  data: Th input; q_PB output; rays input
function q_PB = fcn(Th, rays)
q_PB = quatPB(Th, rays);
end

== matlab function xfl_ukf2/model/dynamic/airforce/air force I ==
  data: r_dot input; f output; ro input; c input; S input
function f = fcn(r_dot, ro, c, S)
f = -ro*c*S*norm(r_dot)*r_dot/2;

== matlab function xfl_ukf2/control/xflControl/Th W/w postpriori ==
  data: Th input; W output; f input; t input; qBI input
function W = fcn(Th, f, t, qBI)

f = quatRotate(quatDual(qBI), f);
R = quat2rotm(qBI');

J = xfl_J_B(Th(1),Th(2),Th(3),Th(4));
J_t = J(4:6, :);
J_f = J(1:3, :);
J_f_I = R * J_f;
A = [J_t; J_f_I(3, :)];

Apinv = pinv(A);
y = [t; f(3)];
W = Apinv*y;

end

== matlab function xfl_ukf2/control/xflControl/Th W/th reg/thdot limit ==
  data: Th_des input; Th0 input; Th output
function Th = fcn(Th_des, Th0)

dt = 1e-2;
K = 12;
dTh1 = (Th_des - Th0);
Th = Th0 + K*dTh1*dt;
end

== matlab function xfl_ukf2/control/xflControl/Th W/dTh lim/thdot limit ==
  data: Th input; Th0 input; Th_limited output; Th_dot output; dt input
function [Th_limited, Th_dot]= fcn(Th, Th0, dt)
lim = 5;
dTh = Th - Th0;
Th_dot = dTh ./ dt;
Th_dot = min(max(Th_dot, - lim), lim);
Th_limited = Th0 + Th_dot * dt;
end

== matlab function xfl_ukf2/control/xflControl/limit q ==
  data: qIn input; q output
function q = fcn(qIn)
eps = 1e-3;
PitchRollLim = 10*pi/180;
eul = quat2eul(qIn');
pr = eul(2:3);
npr = norm(pr);
if norm(npr) < eps
    q = qIn;
else
    pr = PitchRollLim*pr/npr;
    eulLimited = [eul(1) pr];
    q = (eul2quat(eulLimited))';
end
end

== matlab function xfl_ukf2/control/xflControl/Th W/ddTh lim1/thdot limit ==
  data: Th2 input; Th1 input; Th0 input; Th_limited output; dTh1_limited output; dt input; ddTh output
function [Th_limited, dTh1_limited, ddTh]= fcn(Th2, Th1, Th0, dt)

lim = 1;

dTh1 = (Th2 - Th1) / dt;
dTh0 = (Th1 - Th0) / dt;
ddTh = (dTh1 - dTh0) / dt;

ddTh = min(max(ddTh, - lim), lim);
dTh1_limited = dTh0 + ddTh*dt;

Th_limited = Th1 + dTh1_limited * dt + 0.5 * ddTh * dt * dt;
end

== matlab function xfl_ukf2/control/xflControl/Th W1/hyro torque prediction ==
  data: ThDot input; W0 input; t_hyro_predicted output; Ip input
function t_hyro_predicted = fcn(ThDot, W0, Ip)
t_hyro_predicted = zeros(3,1);
angle = 0;
pin = [0;0;1];
for i=1:4
    quatRnToR1 = [cos(angle/2); pin*sin(angle/2)];
    omega = [ThDot(i);0;sign(W0(i))*sqrt(abs(W0(i)))];
     t_hyro_n_Rn = cross(omega, Ip*omega);
     t_hyro_n_R1 = quatRotate(quatRnToR1, t_hyro_n_Rn);
     t_hyro_predicted = t_hyro_predicted + t_hyro_n_R1; 
     angle = angle + pi/2;
end

end

== matlab function xfl_ukf2/UKF/x_apr/X0 ==
  data: x input; X0 output; Px input; gamma input; L input
function X0  = fcn(x, Px, gamma, L)   

L = 13;
X0 = zeros(L, 2*L+1);
X0(:, 1) = x;

sqrtPx = real(sqrtm(Px));
for i = 2 : L + 1
    delta = gamma *  sqrtPx(:, i - 1);
    X0(:, i) = x + delta;
end

for i = L + 2 : 2*L + 1
    delta = gamma* sqrtPx(:, i - L - 1);
    X0(:, i) = x - delta;
end

== matlab function xfl_ukf2/UKF/x_apr/Xk ==
  data: X0 input; U0 input; dt input; xk_minus output; Xk output; Pxk_minus output; L input; w0m input; wim input; R0 input
function [xk_minus, Xk, Pxk_minus] = fcn(X0, U0, dt, L, w0m, wim, R0)

L = 13;

Xk = zeros(L, 2*L + 1);
xk_minus = zeros(L, 1);

for i = 1 : 2*L + 1
    r0 = X0(1:3, i);
    rdot0 = X0(4:6, i);
    q0 = X0(7:10, i);
    omega0 = X0(11:13, i);
    omegaq0 = [0; omega0];
    qdot0 = 0.5*quatMultiply(q0, omegaq0);
    
    rddot = U0(1:3, i);
    omegadot = U0(4:6, i);
    
    r = r0 + rdot0 * dt;
    rdot = rdot0 + rddot * dt;
    q = q0 + qdot0*dt;
    q = q / norm(q);
    omega = omega0 + omegadot * dt;
    Xk(:, i) = [r; rdot; q; omega];
    
    if i == 1
        xk_minus = xk_minus +  w0m * Xk(:, 1);
    else
        xk_minus = xk_minus +  wim * Xk(:, i);
    end
end


wmsumm = w0m;
Pxk_minus = R0;
Pxk_minus = Pxk_minus + w0m*(X0(:, 1) - xk_minus) * (X0(:, 1) - xk_minus)';
for j = 2 : 2*L + 1
        Pxk_minus = Pxk_minus + wim*(X0(:, j) - xk_minus) * (X0(:, j) - xk_minus)';
        wmsumm = wmsumm + wim;
end
wmsumm;

== matlab function xfl_ukf2/control/xflControl/Th W/resolve a priory ==
  data: Th output; f input; W output; t input; T0 input
function [Th, W]= fcn(f, t, T0)
x = [f;t];
%%
tI = 0.5*x(6) + T0;
tII = 0.5*x(6) - T0;

w2 = solutionW2(x(1), x(3)/2, x(4), tII);
th2 = solutionTh2(x(1), x(3)/2, x(4), tII);
w4 = solutionW4(x(1), x(3)/2, x(4), tII);
th4 = solutionTh4(x(1), x(3)/2, x(4), tII);

w1 = solutionW1(x(2), x(3)/2, x(5), tI);
th1 = solutionTh1(x(2), x(3)/2, x(5), tI);
w3 = solutionW3(x(2), x(3)/2, x(5), tI);
th3 = solutionTh3(x(2), x(3)/2, x(5), tI);

W = [w1;w2;w3;w4];
Th = [th1;th2;th3;th4];


% J = xfl_J_B(Th(1),Th(2),Th(3),Th(4));
% xcheck = J*W

end

== matlab function xfl_ukf2/control/xflControl/Th W1/resolve a postpriori ==
  data: Th input; rF input; W output; rT input
function W = fcn(Th, rF, rT)
W = zeros(4,1);

J = xflJ(Th(1),Th(2),Th(3),Th(4));
Jt = J(4:6, :);
eqF = J(3, :);

A = [eqF; Jt];
pA = pinv(A);
y = [rF(3); rT];
W = pA*y;

end

== matlab function xfl_ukf2/control/xflControl/Th W1/resolve a priory ==
  data: Th output; f input; W output; t input; T0 input
function [Th, W]= fcn(f, t, T0)
x = [f;t];
%%
tI = 0.5*x(6) + T0;
tII = 0.5*x(6) - T0;

w2 = solutionW2(x(1), x(3)/2, x(4), tII);
th2 = solutionTh2(x(1), x(3)/2, x(4), tII);
w4 = solutionW4(x(1), x(3)/2, x(4), tII);
th4 = solutionTh4(x(1), x(3)/2, x(4), tII);

w1 = solutionW1(x(2), x(3)/2, x(5), tI);
th1 = solutionTh1(x(2), x(3)/2, x(5), tI);
w3 = solutionW3(x(2), x(3)/2, x(5), tI);
th3 = solutionTh3(x(2), x(3)/2, x(5), tI);

W = [w1;w2;w3;w4];
Th = [th1;th2;th3;th4];


% J = xfl_J_B(Th(1),Th(2),Th(3),Th(4));
% xcheck = J*W

end

== matlab function xfl_ukf2/control/xflControl/Th W1/resolve hyro/resolve hyro ==
  data: W output; Th output; f input; t input; m input; gV input; k input; b input
function [W, Th]= fcn(f, t, m, gV, k, b)
x = [f;t];
g = abs(gV(3));
T0 = m*g*b/2/k;
%%
tI = 0.5*x(6) - T0;
tII = 0.5*x(6) + T0;

w2 = solutionW2(x(1), x(3)/2, x(4), tII);
th2 = solutionTh2(x(1), x(3)/2, x(4), tII);
w4 = solutionW4(x(1), x(3)/2, x(4), tII);
th4 = solutionTh4(x(1), x(3)/2, x(4), tII);

w1 = solutionW1(x(2), x(3)/2, x(5), tI);
th1 = solutionTh1(x(2), x(3)/2, x(5), tI);
w3 = solutionW3(x(2), x(3)/2, x(5), tI);
th3 = solutionTh3(x(2), x(3)/2, x(5), tI);

W = [w1;w2;w3;w4];
Th = [th1;th2;th3;th4];

end

== matlab function xfl_ukf2/UKF/x_apr/xk  ==
  data: xk_minus input; Xk input; Pxk_minus input; xk output; Pxk output; Th input; W input; airdrag_coeff input; m input; g input; yk input; w0c input; wic input; w0m input; wim input; Q input
function [xk, Pxk]= fcn(xk_minus, Xk, Pxk_minus, Th, W, airdrag_coeff, m, g, yk, w0c, wic, w0m, wim, Q)

L = 13;
yN = 13;

Y_minus = zeros(L, 2*L + 1);
yk_minus = zeros(yN, 1);

for i = 1 : 2*L + 1
    r = Xk(1:3, i);
    rdot = Xk(4:6, i);
    qBI = Xk(7:10, i);
    omega = Xk(11:13, i);
    Y_minus(:, i) = [r; rdot; qBI; omega];
    if i == 1
        yk_minus = yk_minus + w0m * Y_minus(:, i);
    else
        yk_minus = yk_minus + wim * Y_minus(:, i);
    end
end


Py = zeros(yN, yN) + Q;
Pxy = zeros(L, yN);
Py = Py + w0m * (Y_minus(:, 1) - yk_minus) * (Y_minus(:, 1) - yk_minus)';
Pxy = Pxy + w0m * (Xk(:, 1) - xk_minus) * (Y_minus(:, 1) - yk_minus)';
for j = 2 : 2*L + 1
    Py = Py + wim * (Y_minus(:, j) - yk_minus) * (Y_minus(:, j) - yk_minus)';
    Pxy = Pxy + wim * (Xk(:, j) - xk_minus) * (Y_minus(:, j) - yk_minus)'; 
end

Py_inversed = Py^-1;
K = Pxy * Py_inversed;
xk = xk_minus + K*(yk - yk_minus);
Pxk = Pxk_minus - K * Py * K';
Pxk = abs(Pxk); %% FIX

== matlab function xfl_ukf2/control/xflControl/Th W1/thdot limit ==
  data: Th input; Th_limited output; Th0 input; Th_dot output; dt input
function [Th_limited, Th_dot]= fcn(Th, Th0, dt)
lim = 10;
dTh = Th - Th0;
Th_dot = dTh/dt;
Th_limited = min(max(Th_dot, - lim), lim);
end

== matlab function xfl_ukf2/control/xflControl/Th W1/toR1 ==
  data: fB input; fR1 output; tB input; tR1 output
function [fR1, tR1]= fcn(fB, tB)
q = [cos(pi/4/2) 0 0 -sin(pi/4/2)]';
fR1 = quatRotate(q, fB);
tR1 = quatRotate(q, tB);
end

== matlab function xfl_ukf2/control/xflControl/regulator/limit course changing/limit course changing ==
  data: x1 input; x output; x0 input
function x = translate(x1, x0)

v1 = x1 .* [1 1 0]';
v0 = x0 .* [1 1 0]';

n_v1 = norm(v1);
n_v0 = norm(v0);
n_lim = 0.5;
if n_v1 < n_lim || n_v0 < n_lim
    v = v1;
else
    v0_n = v0 / n_v0;
    v1_n = v1 / n_v1;
    pin = cross(v1_n, v0_n);
    alpha = norm(cross(v1, v0));

    alpha_lim = pi/8;
    alpha_limited = min(max(-alpha_lim, alpha), alpha_lim);
    q_limited = [cos(alpha_limited/2); -pin * sin(alpha_limited/2)];
    
    v = quatRotate(q_limited, v0);
end

x = [v(1) v(2) x1(3)]';

end

== matlab function xfl_ukf2/sensors/n ==
  data: x input; rHSigma input; y output; rVSigma input
function y = fnc(x, rHSigma, rVSigma)
y  = x + [normrnd(0, rHSigma); normrnd(0, rHSigma); normrnd(0, rVSigma)];
end

== matlab function xfl_ukf2/sensors/n4 ==
  data: x input; A input; y output
function y = fnc(x, A)
y  = x + [normrnd(0, A); normrnd(0, A); normrnd(0, A)];
end

== matlab function xfl_ukf2/control/xflControl/regulator/req_moment ==
  data: q_reg input; req_moment output; I_B input
function req_moment = translate(q_reg, I_B)
req_moment = I_B*q_reg;
end

== matlab function xfl_ukf2/UKF/norm1 ==
  data: q input; qn output
function qn = fcn(q)
qn = q/norm(q);
end

== matlab function xfl_ukf2/UKF/norm3 ==
  data: q input; qn output
function qn = fcn(q)
qn = q/norm(q);
end

== matlab function xfl_ukf2/UKF/r2eul ==
  data: q input; x output
function x = fnc(q)
eul = quat2eul(q');
x = eul';
end

== matlab function xfl_ukf2/sensors/n1 ==
  data: x input; A input; y output
function y = fnc(x, A)
y  = x + [normrnd(0, A); normrnd(0, A); normrnd(0, A)];
end

== matlab function xfl_ukf2/UKF/x_apr/dyn model/simple model ==
  data: Th input; W input; Xs input; U0 output; m input; g input; I input; airdrag_coeff input
function U0 = q2R(Th, W, Xs, m, g, I, airdrag_coeff)
J = xfl_J_B(Th(1),Th(2),Th(3),Th(4));
xdyn = J*W;
F = xdyn(1:3);
tau = xdyn(4:6);

sizeXs = size(Xs);
L = 2*sizeXs(1) + 1;

U0 = zeros(6, L);
for i = 1 : L
    qBI = Xs(7:10, i);
    rdot = Xs(4:6, i);
    omega = Xs(11:13, i);
    U0(1:3, i) = (quatRotate(qBI, F) + 0*airdrag_coeff*norm(rdot)*rdot + m*g)/m;
    U0(4:6, i) = I^-1 * (tau - cross(omega, I * omega));
end

== matlab function xfl_ukf2/control/xflControl/regulator/req_force_I ==
  data: r_reg input; req_force_I output; m input; gN input
function req_force_I = translate(r_reg, m, gN)
req_force_I = m*r_reg + [0;0;1]*m*gN;
end

== matlab function xfl_ukf2/sensors/q > eul + eulNoise > q ==
  data: q input; roll_pitch_sigma input; q_out output; yaw_sigma input
function q_out = fnc(q, roll_pitch_sigma, yaw_sigma)

eul = quat2Eul(q);
eul(1) = eul(1) + normrnd(0, roll_pitch_sigma);
eul(2) = eul(2) + normrnd(0, roll_pitch_sigma);
eul(3) = eul(3) + normrnd(0, yaw_sigma);
q_out = quatFromEul(eul);

end

== matlab function xfl_ukf2/sensors/n3 ==
  data: x input; density input; y output; bias input; dt input; bias_accumulated0 input; bias_accumulated output
function [y, bias_accumulated]= fnc(x, density, bias, dt, bias_accumulated0)
bias_accumulated = bias_accumulated0 + normrnd(bias * dt, bias * dt/10);
y = x + [normrnd(0, sqrt(density)); normrnd(0, sqrt(density)); normrnd(0, sqrt(density))] + bias_accumulated;
end

== matlab function xfl_ukf2/control/xflControl/toI ==
  data: fB input; fI output; qBI input
function fI = q2R(fB, qBI)
qIB = quatDual(qBI);
fI = quatRotate(qBI, fB);
end
